simulink model "BiT_Simulation"  (R2025b)
settings: Solver=VariableStepAuto  StartTime=0.0  StopTime=11  RelTol=1e-3
model workspace (MAT data in the model file):
  alpha1 = 0.0546520983298
  alpha2 = 0.559430927786
  alpha3 = 9.81
  k_w = 28
  tau_w = 1.6
values from neighbouring files (symbols this model uses):
  Init_cond = [0.0; 0; w_0]    [Ball_in_Tube.m]    (also in Ball_in_Tube_toggling.m)
  Kd = 1.118    [Ball_in_Tube.m]    (also in Ball_in_Tube_toggling.m)
  Ki = 0.5    [Ball_in_Tube.m]    (also in Ball_in_Tube_toggling.m)
  Kp = 1.5    [Ball_in_Tube.m]    (also in Ball_in_Tube_toggling.m)
  LowerLim = [0; -100; 0]    [Ball_in_Tube.m]    (also in Ball_in_Tube_toggling.m)
  UpperLim = [0.35; 100; 200]    [Ball_in_Tube.m]    (also in Ball_in_Tube_toggling.m)
libraries: simulink x1, slpidlib x1
settings Model: Creator=busoj  LastModifiedBy=Felix

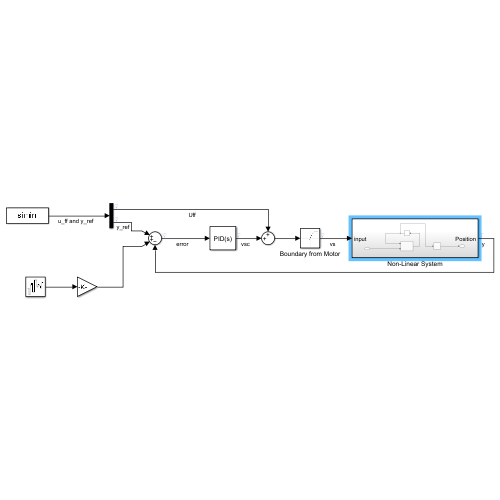
[thumbnail: Simulink's stored preview of the top-level diagram]
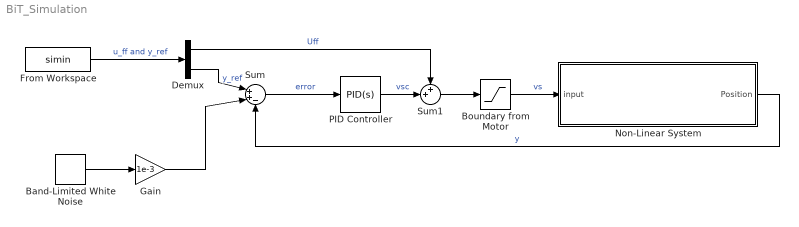
== system BiT_Simulation ==
  Band-Limited White Noise : simulink/Sources/Band-Limited White Noise  Cov=[0.1]  Ts=0.1  seed=[23341]
  Boundary from Motor : Saturate  UpperLimit=5  LowerLimit=0
  Demux : Demux  Outputs=2
  From Workspace : FromWorkspace  VariableName=simin
  Gain : Gain  Gain=1e-3
  Non-Linear System : Subsystem
  PID Controller : slpidlib/PID Controller  Controller=PID  Form=Parallel  TimeDomain=Continuous-time  UseExternalTs=off  SampleTime=-1  IntegratorMethod=Forward Euler  FilterMethod=Forward Euler  ControllerParametersSource=internal  P=Kp  I=Ki  UseKiTs=off  D=Kd  UseExternalDerivativeSource=off  N=100  UseFilter=on  TunerSelectOption=Transfer Function Based (PID Tuner App)  InitialConditionSource=internal  InitialConditionForIntegrator=0  InitialConditionForFilter=0  DifferentiatorICPrevScaledInput=0  ExternalReset=none  TrackingMode=off  Kt=1  LimitOutput=off  SatLimitsSource=internal  UpperSaturationLimit=inf  LowerSaturationLimit=-inf  LinearizeAsGain=on  AntiWindupMode=none  Kb=1  LimitIntegrator=off  UpperIntegratorSaturationLimit=inf  LowerIntegratorSaturationLimit=-inf  POutMin=[]  POutMax=[]  IOutMin=[]  IOutMax=[]  DOutMin=[]  DOutMax=[]  NOutMin=[]  NOutMax=[]  SumOutMin=[]  SumOutMax=[]  SaturationOutMin=[]  SaturationOutMax=[]  PParamMin=[]  PParamMax=[]  IParamMin=[]  IParamMax=[]  DParamMin=[]  DParamMax=[]  NParamMin=[]  NParamMax=[]  KbParamMin=[]  KbParamMax=[]  KtParamMin=[]  KtParamMax=[]  KbOutMin=[]  KbOutMax=[]  KtOutMin=[]  KtOutMax=[]  IntegratorOutMin=[]  IntegratorOutMax=[]  FilterOutMin=[]  FilterOutMax=[]  SumI1OutMin=[]  SumI1OutMax=[]  SumI2OutMin=[]  SumI2OutMax=[]  SumI3OutMin=[]  SumI3OutMax=[]  SumI4OutMin=[]  SumI4OutMax=[]  SumDOutMin=[]  SumDOutMax=[]  DifferentiatorOutMin=[]  DifferentiatorOutMax=[]  FilterDiffOutCoefMin=[]  FilterDiffOutCoefMax=[]  ReciprocalOutMin=[]  ReciprocalOutMax=[]  SumDenOutMin=[]  SumDenOutMax=[]  SumNumOutMin=[]  SumNumOutMax=[]  DivideOutMin=[]  DivideOutMax=[]  UdiffTsProdOutMin=[]  UdiffTsProdOutMax=[]  NTsProdOutMin=[]  NTsProdOutMax=[]  UintegralTsProdOutMin=[]  UintegralTsProdOutMax=[]  UngainTsProdOutMin=[]  UngainTsProdOutMax=[]  ClampingZeroOutDataTypeStr=Inherit: Inherit via back propagation  ClampingZeroOutMin=[]  ClampingZeroOutMax=[]  FilterDenConstantOutDataTypeStr=Inherit: Inherit via back propagation  FilterDenConstantOutMin=[]  FilterDenConstantOutMax=[]  PCopyOutDataTypeStr=Inherit: Inherit via back propagation  PCopyOutMin=[]  PCopyOutMax=[]  NCopyOutDataTypeStr=Inherit: Inherit via back propagation  NCopyOutMin=[]  NCopyOutMax=[]  IntegratorContinuousStateAttributes=''  IntegratorStateMustResolveToSignalObject=off  IntegratorRTWStateStorageClass=Auto  FilterContinuousStateAttributes=''  FilterStateMustResolveToSignalObject=off  FilterRTWStateStorageClass=Auto  ParallelPVariant=InternalParameters  IdealPVariant=Disabled  IVariant=InternalParameters  DVariant=InternalParameters  IntegratorVariant=Continuous  SatVariant=Disabled  AWVariant=Passthrough  PCopyVariant=Disabled  TRVariant=Disabled  FdbkBlocksVariant=Forward  IdealPFdbkVariant=Disabled  SatFdbkVariant=Disabled  DerivativeFilterVariant=ContFilter  NVariant=InternalParameters  NCopyVariant=Disabled  FilterICVariant=InternalICsFilter  IntegratorICVariant=InternalICs  ExternalResetVariant=Disabled  TRSumVariant=Passthrough  SumFdbkVariant=Disabled  SumVariant=Sum_PID  TsampFilterVariant=InternalTs  TsampNgainVariant=Passthrough  TsampIntegralVariant=Disabled_SignalSpec  ExternalSaturationOutDataTypeStr=Inherit: Same as second input  DerivativeSourceVariant=ErrorSignal  PreIntVariant=InternalPreInt
  Sum : Sum  Inputs=|++-
  Sum1 : Sum  Inputs=++|
  wires:
  Sum/1 -> PID Controller/1  "error"
  Band-Limited White Noise/1 -> Gain/1
  From Workspace/1 -> Demux/1  "u_ff and y_ref"
  Demux/2 -> Sum/1  "y_ref"
  Demux/1 -> Sum1/1  "Uff"
  Sum1/1 -> Boundary from Motor/1
  Boundary from Motor/1 -> Non-Linear System/1(input)  "vs"
  PID Controller/1 -> Sum1/2  "vsc"
  Gain/1 -> Sum/2
  Non-Linear System/1(Position) -> Sum/3  "y"

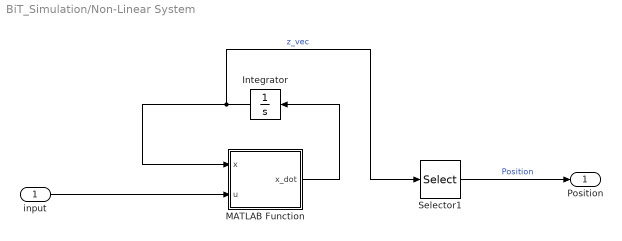
== system BiT_Simulation/Non-Linear System ==
  input : Inport
  Integrator : Integrator  InitialCondition=Init_cond  UpperSaturationLimit=UpperLim  LowerSaturationLimit=LowerLim
  MATLAB Function : MATLAB Function  TreatAsAtomicUnit=on
  Selector1 : Selector  InputPortWidth=3  IndexOptions=Index vector (dialog)  Indices=1  OutputSizes=1
  Position : Outport
  wires:
  MATLAB Function/1(x_dot) -> Integrator/1
  Integrator/1 -> Selector1/1, MATLAB Function/1(x)  "z_vec"
  input/1 -> MATLAB Function/2(u)
  Selector1/1 -> Position/1  "Position"

== matlab function BiT_Simulation/Non-Linear System/MATLAB Function ==
  data: x_dot output; x input; u input; alpha1 parameter; alpha2 parameter; alpha3 parameter; tau_w parameter; k_w parameter
function x_dot  = fcn(x, u, alpha1, alpha2, alpha3, tau_w, k_w)

A_NL = [x(2); (alpha1*x(3) - alpha2*x(2))^2 - alpha3; -(1/tau_w)*x(3)];
b_NL = [0; 0; k_w/tau_w];

x_dot = A_NL + b_NL*u;
% y = x;
